simulink model "trescinco"  (R2015a)
settings: Solver=ode45  StartTime=0.0  StopTime=1000  RelTol=1e-3
settings Model: Creator=Diogo  LastModifiedBy=Alunos

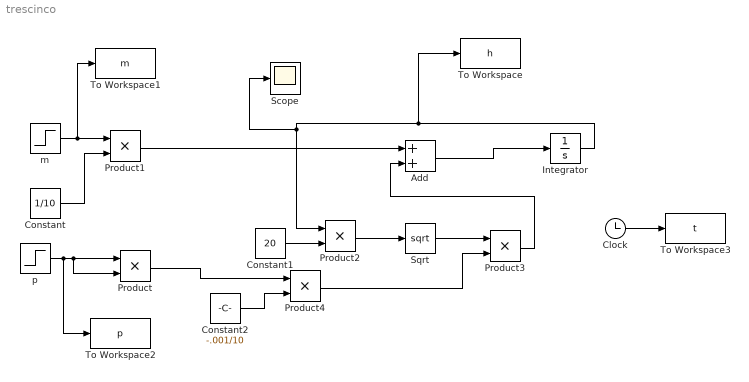
== system trescinco ==
  Add : Sum
  Clock : Clock
  Constant : Constant  Value=1/10
  Constant1 : Constant  Value=20
  Constant2 : Constant  Value=-.001/10
  Integrator : Integrator  InitialCondition=5
  Product{,1..4} (5 alike) : Product
  Scope : Scope
  Sqrt : Sqrt  SaturateOnIntegerOverflow=on
  To Workspace : ToWorkspace  VariableName=h  SampleTime=-1
  To Workspace1 : ToWorkspace  VariableName=m  SampleTime=-1
  To Workspace2 : ToWorkspace  VariableName=p  SampleTime=-1
  To Workspace3 : ToWorkspace  VariableName=t  SampleTime=-1
  m : Step  Before=1  SampleTime=0
  p : Step  Before=10  After=10.1  SampleTime=0
  wires:
  m/1 -> To Workspace1/1, Product1/1
  Constant/1 -> Product1/2
  p/1 -> To Workspace2/1, Product/2, Product/1
  Constant1/1 -> Product2/2
  Integrator/1 -> To Workspace/1, Scope/1, Product2/1
  Product2/1 -> Sqrt/1
  Sqrt/1 -> Product3/1
  Product/1 -> Product4/1
  Constant2/1 -> Product4/2
  Product4/1 -> Product3/2
  Product3/1 -> Add/2
  Product1/1 -> Add/1
  Add/1 -> Integrator/1
  Clock/1 -> To Workspace3/1
